simulink model "controller"  (R2019b)
settings: Solver=FixedStepDiscrete  StartTime=0.0  StopTime=10.0  FixedStep=0.01  RelTol=1e-3
settings Model: Creator=dommaschkj  LastModifiedBy=ReinfeldR
settings DataIOCC: ReturnWorkspaceOutputs=off
settings OptimizationCC: DefaultParameterBehavior=Inlined  UseDivisionForNetSlopeComputation=on  PassReuseOutputArgsAs=Individual arguments  MaxStackSize=64  EfficientTunableParamExpr=on
settings DebuggingCC: SignalInfNanChecking=warning  IntegerOverflowMsg=error  ParameterTunabilityLossMsg=error  AssertControl=DisableAll  SFUndirectedBroadcastEventsDiag=error  ArithmeticOperatorsInVariantConditions=warning
settings HardwareCC: ProdBitPerPointer=32  ProdBitPerSizeT=32  ProdBitPerPtrDiffT=32  ProdLargestAtomicInteger=LongLong  ProdLargestAtomicFloat=Double  ProdWordSize=32  ProdLongLongMode=on  ProdHWDeviceType=Custom Processor->Custom Processor
settings SFSimCC: SimUseLocalCustomCode=off  CompileTimeRecursionLimit=0  EnableRuntimeRecursion=off  MATLABDynamicMemAlloc=off  CustomCodeUndefinedFunction=UseInterfaceOnly
settings RTWCC: SystemTargetFile=ert.tlc  GenCodeOnly=on  PackageGeneratedCodeAndArtifacts=on  PackageName=controller  TemplateMakefile=ert_default_tmf  GenerateReport=on  RTWUseLocalCustomCode=off  Toolchain=GNU Tools for ARM Embedded Processors  IncludeHyperlinkInReport=on  LaunchReport=on  TargetLang=C++  GenerateTraceInfo=on  GenerateTraceReport=on  GenerateTraceReportSl=on  GenerateTraceReportSf=on  GenerateTraceReportEml=on
settings CodeAppCC: ForceParamTrailComments=on  IgnoreCustomStorageClasses=off  OperatorAnnotations=on  SimulinkDataObjDesc=on  SFDataObjDesc=on  MATLABFcnDesc=on  InsertBlockDesc=on
settings ERTTargetCC: TargetLangStandard=C99 (ISO)  UtilityFuncGeneration=Shared location  MultiwordLength=64  MultiInstanceERTCode=on  CodeInterfacePackaging=C++ class  SupportNonFinite=off  SupportComplex=off  ParenthesesLevel=Maximum  CastingMode=Standards  GenerateSharedConstants=off  InlinedParameterPlacement=NonHierarchical  RootIOFormat=Structure reference  ERTCustomFileTemplate=example_file_process.tlc  ERTFilePackagingFormat=Compact  EnableSignedLeftShifts=off  EnableSignedRightShifts=off

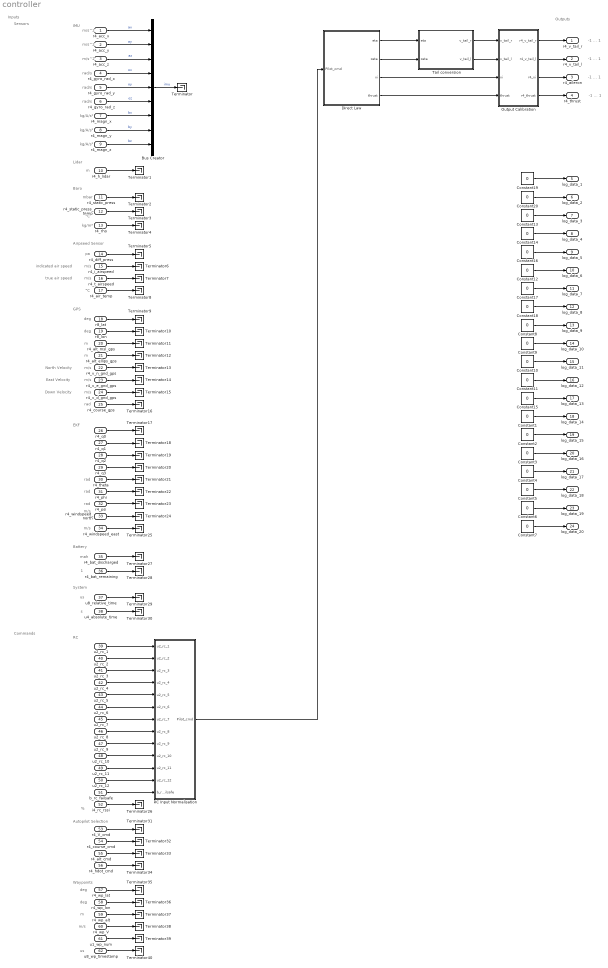
== system controller ==
  note: Sensors
  note: °C
  note: rad
  note: GPS
  note: IMU
  note: °C
  note: deg
  note: -1 ... 1
  note: Lidar
  note: -1 ... 1
  note: pa
  note: m
  note: m/s
  note: Down Velocity
  note: m
  note: North Velocity
  note: East Velocity
  note: m
  note: m/s^2
  note: Inputs
  note: -1 ... 1
  note: m/s
  note: -1 ... 1
  note: m/s
  note: m/s^2
  note: Outputs
  note: Airpseed Sensor
  note: mbar
  note: deg
  note: EKF
  note: rad
  note: Baro
  note: rad
  note: true air speed
  note: m/s^2
  note: rad
  note: m/s
  note: Battery
  note: kg/m³
  note: rad/s
  note: rad/s
  note: rad/s
  note: kg/A/s²
  note: kg/A/s²
  note: kg/A/s²
  note: m/s
  note: indicated air speed
  note: m/s
  note: m/s
  note: mah
  note: 1
  note: %
  note: us
  note: s
  note: System
  note: RC
  note: Commands
  note: Autopilot Selection
  note: Waypoints
  note: deg
  note: m
  note: m/s
  note: deg
  note: us
  r4_acc_x : Inport  OutDataTypeStr=single  Unit=m/s^2  PortDimensions=1  SampleTime=1/100  Interpolate=off
  r4_acc_y : Inport  Port=2  OutDataTypeStr=single  Unit=m/s^2  PortDimensions=1  SampleTime=1/100  Interpolate=off
  r4_acc_z : Inport  Port=3  OutDataTypeStr=single  Unit=m/s^2  PortDimensions=1  SampleTime=1/100  Interpolate=off
  r4_gyro_rad_x : Inport  Port=4  OutDataTypeStr=single  Unit=rad/s  PortDimensions=1  SampleTime=1/100  Interpolate=off
  r4_gyro_rad_y : Inport  Port=5  OutDataTypeStr=single  Unit=rad/s  PortDimensions=1  SampleTime=1/100  Interpolate=off
  r4_gyro_rad_z : Inport  Port=6  OutDataTypeStr=single  Unit=rad/s  PortDimensions=1  SampleTime=1/100  Interpolate=off  LockScale=on
  r4_magn_x : Inport  Port=7  OutDataTypeStr=single  Unit=kg/A/s^2  PortDimensions=1  SampleTime=1/100  Interpolate=off
  r4_magn_y : Inport  Port=8  OutDataTypeStr=single  Unit=kg/A/s^2  PortDimensions=1  SampleTime=1/100  Interpolate=off
  r4_magn_z : Inport  Port=9  OutDataTypeStr=single  Unit=kg/A/s^2  PortDimensions=1  SampleTime=1/100  Interpolate=off
  r4_h_lidar : Inport  Port=10  OutDataTypeStr=single  Unit=m  PortDimensions=1  SampleTime=1/100  Interpolate=off
  r4_static_press : Inport  Port=11  OutDataTypeStr=single  Unit=mbar  PortDimensions=1  SampleTime=1/100  Interpolate=off
  r4_static_press_temp : Inport  Port=12  OutDataTypeStr=single  Unit=°C  PortDimensions=1  SampleTime=1/100  Interpolate=off
  r4_rho : Inport  Port=13  OutDataTypeStr=single  Unit=kg/m^3  PortDimensions=1  SampleTime=1/100  Interpolate=off
  r4_diff_press : Inport  Port=14  OutDataTypeStr=single  Unit=Pa  PortDimensions=1  SampleTime=1/100  Interpolate=off
  r4_i_airspeed : Inport  Port=15  OutDataTypeStr=single  Unit=m/s  PortDimensions=1  SampleTime=1/100  Interpolate=off
  r4_t_airspeed : Inport  Port=16  OutDataTypeStr=single  Unit=m/s  PortDimensions=1  SampleTime=1/100  Interpolate=off
  r4_air_temp : Inport  Port=17  OutDataTypeStr=single  Unit=°C  PortDimensions=1  SampleTime=1/100  Interpolate=off
  r8_lat : Inport  Port=18  OutDataTypeStr=double  Unit=deg  PortDimensions=1  SampleTime=1/2  Interpolate=off
  r8_lon : Inport  Port=19  OutDataTypeStr=double  Unit=deg  PortDimensions=1  SampleTime=1/2  Interpolate=off
  r4_alt_msl_gps : Inport  Port=20  OutDataTypeStr=single  Unit=m  PortDimensions=1  SampleTime=1/2  Interpolate=off
  r4_alt_ellips_gps : Inport  Port=21  OutDataTypeStr=single  Unit=m  PortDimensions=1  SampleTime=1/2  Interpolate=off
  r4_v_n_gnd_gps : Inport  Port=22  OutDataTypeStr=single  Unit=m/s  PortDimensions=1  SampleTime=1/2  Interpolate=off
  r4_v_e_gnd_gps : Inport  Port=23  OutDataTypeStr=single  Unit=m/s  PortDimensions=1  SampleTime=1/2  Interpolate=off
  r4_v_d_gnd_gps : Inport  Port=24  OutDataTypeStr=single  Unit=m/s  PortDimensions=1  SampleTime=1/2  Interpolate=off
  r4_course_gps : Inport  Port=25  OutDataTypeStr=single  Unit=rad  PortDimensions=1  SampleTime=1/2  Interpolate=off
  r4_q0 : Inport  Port=26  OutMin=[-1]  OutMax=[1]  OutDataTypeStr=single  Unit=1  PortDimensions=1  SampleTime=1/100  Interpolate=off
  r4_q1 : Inport  Port=27  OutMin=[-1]  OutMax=[1]  OutDataTypeStr=single  Unit=1  PortDimensions=1  SampleTime=1/100  Interpolate=off
  r4_q2 : Inport  Port=28  OutMin=[-1]  OutMax=[1]  OutDataTypeStr=single  Unit=1  PortDimensions=1  SampleTime=1/100  Interpolate=off
  r4_q3 : Inport  Port=29  OutMin=[-1]  OutMax=[1]  OutDataTypeStr=single  Unit=one  PortDimensions=1  SampleTime=1/100  Interpolate=off
  r4_theta : Inport  Port=30  OutDataTypeStr=single  Unit=rad  PortDimensions=1  SampleTime=1/100  Interpolate=off
  r4_phi : Inport  Port=31  OutDataTypeStr=single  Unit=rad  PortDimensions=1  SampleTime=1/100  Interpolate=off
  r4_psi : Inport  Port=32  OutDataTypeStr=single  Unit=rad  PortDimensions=1  SampleTime=1/100  Interpolate=off
  r4_windspeed_north : Inport  Port=33  OutDataTypeStr=single  Unit=m/s  PortDimensions=1  SampleTime=1/100  Interpolate=off
  r4_windspeed_east : Inport  Port=34  OutDataTypeStr=single  Unit=m/s  PortDimensions=1  SampleTime=1/100  Interpolate=off
  r4_bat_discharged : Inport  Port=35  OutDataTypeStr=single  Unit=mA*hr  PortDimensions=1  SampleTime=1/100  Interpolate=off
  r4_bat_remaining : Inport  Port=36  OutDataTypeStr=single  PortDimensions=1  SampleTime=1/100  Interpolate=off
  u8_relative_time : Inport  Port=37  OutDataTypeStr=uint64  Unit=µs  PortDimensions=1  SampleTime=1/100  Interpolate=off
  u4_absolute_time : Inport  Port=38  OutDataTypeStr=uint32  Unit=s  PortDimensions=1  SampleTime=1/100  Interpolate=off
  u2_rc_1 : Inport  Port=39  OutDataTypeStr=uint16  PortDimensions=1  SampleTime=1/100  Interpolate=off
  u2_rc_2 : Inport  Port=40  OutDataTypeStr=uint16  PortDimensions=1  SampleTime=1/100  Interpolate=off
  u2_rc_3 : Inport  Port=41  OutDataTypeStr=uint16  PortDimensions=1  SampleTime=1/100  Interpolate=off
  u2_rc_4 : Inport  Port=42  OutDataTypeStr=uint16  PortDimensions=1  SampleTime=1/100  Interpolate=off
  u2_rc_5 : Inport  Port=43  OutDataTypeStr=uint16  PortDimensions=1  SampleTime=1/100  Interpolate=off
  u2_rc_6 : Inport  Port=44  OutDataTypeStr=uint16  PortDimensions=1  SampleTime=1/100  Interpolate=off
  u2_rc_7 : Inport  Port=45  OutDataTypeStr=uint16  PortDimensions=1  SampleTime=1/100  Interpolate=off
  u2_rc_8 : Inport  Port=46  OutDataTypeStr=uint16  PortDimensions=1  SampleTime=1/100  Interpolate=off
  u2_rc_9 : Inport  Port=47  OutDataTypeStr=uint16  PortDimensions=1  SampleTime=1/100  Interpolate=off
  u2_rc_10 : Inport  Port=48  OutDataTypeStr=uint16  PortDimensions=1  SampleTime=1/100  Interpolate=off
  u2_rc_11 : Inport  Port=49  OutDataTypeStr=uint16  PortDimensions=1  SampleTime=1/100  Interpolate=off
  u2_rc_12 : Inport  Port=50  OutDataTypeStr=uint16  PortDimensions=1  SampleTime=1/100  Interpolate=off
  b_rc_failsafe : Inport  Port=51  OutDataTypeStr=boolean  PortDimensions=1  SampleTime=1/100  Interpolate=off
  i4_rc_rssi : Inport  Port=52  OutDataTypeStr=int32  PortDimensions=1  SampleTime=1/100  Interpolate=off
  r4_V_cmd : Inport  Port=53  OutDataTypeStr=single  PortDimensions=1  SampleTime=1/100  Interpolate=off
  r4_course_cmd : Inport  Port=54  OutDataTypeStr=single  PortDimensions=1  SampleTime=1/100  Interpolate=off
  r4_alt_cmd : Inport  Port=55  OutDataTypeStr=single  PortDimensions=1  SampleTime=1/100  Interpolate=off
  r4_hdot_cmd : Inport  Port=56  OutDataTypeStr=single  PortDimensions=1  SampleTime=1/100  Interpolate=off
  r4_wp_lat : Inport  Port=57  OutDataTypeStr=single  Unit=deg  PortDimensions=15  SampleTime=1/100  Interpolate=off
  r4_wp_lon : Inport  Port=58  OutDataTypeStr=single  Unit=deg  PortDimensions=15  SampleTime=1/100  Interpolate=off
  r4_wp_alt : Inport  Port=59  OutDataTypeStr=single  Unit=m  PortDimensions=15  SampleTime=1/100  Interpolate=off
  r4_wp_V : Inport  Port=60  OutDataTypeStr=single  Unit=m/s  PortDimensions=15  SampleTime=1/100  Interpolate=off
  u1_wp_num : Inport  Port=61  OutDataTypeStr=uint8  PortDimensions=1  SampleTime=1/100  Interpolate=off
  u8_wp_timestamp : Inport  Port=62  OutMin=0  OutMax=18446744073709551615  OutDataTypeStr=uint64  Unit=µs  PortDimensions=1  SampleTime=1/100  Interpolate=off
  Bus Creator : BusCreator  Inputs=9
  Constant{1..20} (20 alike) : Constant  Value=0  OutDataTypeStr=single
  Direct Law : Subsystem
  Output Calibration : Subsystem
  RC Input Normalisation : Subsystem
  Tail conversion : Subsystem
  Terminator{,1..40} (41 alike) : Terminator
  r4_v_tail_r : Outport  OutDataTypeStr=single  VectorParamsAs1DForOutWhenUnconnected=off
  r4_v_tail_l : Outport  Port=2  OutDataTypeStr=single  VectorParamsAs1DForOutWhenUnconnected=off
  r4_aileron : Outport  Port=3  OutDataTypeStr=single  VectorParamsAs1DForOutWhenUnconnected=off
  r4_thrust : Outport  Port=4  OutDataTypeStr=single  VectorParamsAs1DForOutWhenUnconnected=off
  log_data_1 : Outport  Port=5  OutDataTypeStr=single  VectorParamsAs1DForOutWhenUnconnected=off
  log_data_2 : Outport  Port=6  OutDataTypeStr=single  VectorParamsAs1DForOutWhenUnconnected=off
  log_data_3 : Outport  Port=7  OutDataTypeStr=single  VectorParamsAs1DForOutWhenUnconnected=off
  log_data_4 : Outport  Port=8  OutDataTypeStr=single  VectorParamsAs1DForOutWhenUnconnected=off
  log_data_5 : Outport  Port=9  OutDataTypeStr=single  VectorParamsAs1DForOutWhenUnconnected=off
  log_data_6 : Outport  Port=10  OutDataTypeStr=single  VectorParamsAs1DForOutWhenUnconnected=off
  log_data_7 : Outport  Port=11  OutDataTypeStr=single  VectorParamsAs1DForOutWhenUnconnected=off
  log_data_8 : Outport  Port=12  OutDataTypeStr=single  VectorParamsAs1DForOutWhenUnconnected=off
  log_data_9 : Outport  Port=13  OutDataTypeStr=single  VectorParamsAs1DForOutWhenUnconnected=off
  log_data_10 : Outport  Port=14  OutDataTypeStr=single  VectorParamsAs1DForOutWhenUnconnected=off
  log_data_11 : Outport  Port=15  OutDataTypeStr=single  VectorParamsAs1DForOutWhenUnconnected=off
  log_data_12 : Outport  Port=16  OutDataTypeStr=single  VectorParamsAs1DForOutWhenUnconnected=off
  log_data_13 : Outport  Port=17  OutDataTypeStr=single  VectorParamsAs1DForOutWhenUnconnected=off
  log_data_14 : Outport  Port=18  OutDataTypeStr=single  VectorParamsAs1DForOutWhenUnconnected=off
  log_data_15 : Outport  Port=19  OutDataTypeStr=single  VectorParamsAs1DForOutWhenUnconnected=off
  log_data_16 : Outport  Port=20  OutDataTypeStr=single  VectorParamsAs1DForOutWhenUnconnected=off
  log_data_17 : Outport  Port=21  OutDataTypeStr=single  VectorParamsAs1DForOutWhenUnconnected=off
  log_data_18 : Outport  Port=22  OutDataTypeStr=single  VectorParamsAs1DForOutWhenUnconnected=off
  log_data_19 : Outport  Port=23  OutDataTypeStr=single  VectorParamsAs1DForOutWhenUnconnected=off
  log_data_20 : Outport  Port=24  OutDataTypeStr=single  VectorParamsAs1DForOutWhenUnconnected=off
  wires:
  Output Calibration/4(r4_thrust) -> r4_thrust/1
  Output Calibration/1(r4_v_tail_r) -> r4_v_tail_r/1
  Output Calibration/3(r4_xi) -> r4_aileron/1
  Output Calibration/2(r4_v_tail_l) -> r4_v_tail_l/1
  Tail conversion/1(v_tail_r) -> Output Calibration/1(v_tail_r)
  Tail conversion/2(v_tail_l) -> Output Calibration/2(v_tail_l)
  Direct Law/4(thrust) -> Output Calibration/4(thrust)
  u2_rc_1/1 -> RC Input Normalisation/1(u2_rc_1)
  u2_rc_2/1 -> RC Input Normalisation/2(u2_rc_2)
  u2_rc_3/1 -> RC Input Normalisation/3(u2_rc_3)
  u2_rc_4/1 -> RC Input Normalisation/4(u2_rc_4)
  u2_rc_5/1 -> RC Input Normalisation/5(u2_rc_5)
  u2_rc_7/1 -> RC Input Normalisation/7(u2_rc_7)
  u2_rc_8/1 -> RC Input Normalisation/8(u2_rc_8)
  u2_rc_6/1 -> RC Input Normalisation/6(u2_rc_6)
  b_rc_failsafe/1 -> RC Input Normalisation/13(b_rc_failsafe)
  Direct Law/3(xi) -> Output Calibration/3(xi)
  Direct Law/2(zeta) -> Tail conversion/2(zeta)
  Direct Law/1(eta) -> Tail conversion/1(eta)
  Bus Creator/1 -> Terminator/1  "imu"
  r4_acc_x/1 -> Bus Creator/1  "ax"
  r4_acc_y/1 -> Bus Creator/2  "ay"
  r4_acc_z/1 -> Bus Creator/3  "az"
  r4_gyro_rad_x/1 -> Bus Creator/4  "ox"
  r4_gyro_rad_y/1 -> Bus Creator/5  "oy"
  r4_gyro_rad_z/1 -> Bus Creator/6  "oz"
  r4_magn_x/1 -> Bus Creator/7  "bx"
  r4_magn_y/1 -> Bus Creator/8  "by"
  r4_magn_z/1 -> Bus Creator/9  "bz"
  r4_h_lidar/1 -> Terminator1/1
  r4_static_press/1 -> Terminator2/1
  r4_static_press_temp/1 -> Terminator3/1
  r4_rho/1 -> Terminator4/1
  r4_diff_press/1 -> Terminator5/1
  r4_i_airspeed/1 -> Terminator6/1
  r4_t_airspeed/1 -> Terminator7/1
  r4_air_temp/1 -> Terminator8/1
  r4_alt_msl_gps/1 -> Terminator11/1
  r4_alt_ellips_gps/1 -> Terminator12/1
  r4_v_n_gnd_gps/1 -> Terminator13/1
  r4_v_e_gnd_gps/1 -> Terminator14/1
  r4_v_d_gnd_gps/1 -> Terminator15/1
  r4_course_gps/1 -> Terminator16/1
  r4_q0/1 -> Terminator17/1
  r4_q1/1 -> Terminator18/1
  r4_q2/1 -> Terminator19/1
  r4_q3/1 -> Terminator20/1
  r4_theta/1 -> Terminator21/1
  r4_phi/1 -> Terminator22/1
  r4_psi/1 -> Terminator23/1
  r4_windspeed_north/1 -> Terminator24/1
  r4_windspeed_east/1 -> Terminator25/1
  i4_rc_rssi/1 -> Terminator26/1
  r4_bat_discharged/1 -> Terminator27/1
  r4_bat_remaining/1 -> Terminator28/1
  u8_relative_time/1 -> Terminator29/1
  u4_absolute_time/1 -> Terminator30/1
  u2_rc_9/1 -> RC Input Normalisation/9(u2_rc_9)
  u2_rc_10/1 -> RC Input Normalisation/10(u2_rc_10)
  u2_rc_11/1 -> RC Input Normalisation/11(u2_rc_11)
  u2_rc_12/1 -> RC Input Normalisation/12(u2_rc_12)
  RC Input Normalisation/1(Pilot_cmd) -> Direct Law/1(Pilot_cmd)
  Constant10/1 -> log_data_11/1
  Constant11/1 -> log_data_12/1
  Constant8/1 -> log_data_9/1
  Constant9/1 -> log_data_10/1
  r4_alt_cmd/1 -> Terminator33/1
  r4_course_cmd/1 -> Terminator32/1
  r4_hdot_cmd/1 -> Terminator34/1
  r4_V_cmd/1 -> Terminator31/1
  Constant15/1 -> log_data_13/1
  Constant2/1 -> log_data_15/1
  Constant4/1 -> log_data_17/1
  Constant1/1 -> log_data_14/1
  Constant5/1 -> log_data_18/1
  Constant7/1 -> log_data_20/1
  Constant3/1 -> log_data_16/1
  Constant6/1 -> log_data_19/1
  Constant20/1 -> log_data_2/1
  Constant14/1 -> log_data_4/1
  Constant18/1 -> log_data_8/1
  Constant19/1 -> log_data_1/1
  Constant17/1 -> log_data_7/1
  Constant13/1 -> log_data_3/1
  Constant12/1 -> log_data_6/1
  Constant16/1 -> log_data_5/1
  r8_lat/1 -> Terminator9/1
  r8_lon/1 -> Terminator10/1
  r4_wp_alt/1 -> Terminator37/1
  r4_wp_V/1 -> Terminator38/1
  r4_wp_lat/1 -> Terminator35/1
  r4_wp_lon/1 -> Terminator36/1
  u8_wp_timestamp/1 -> Terminator40/1
  u1_wp_num/1 -> Terminator39/1

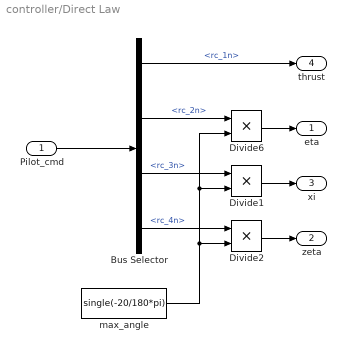
== system controller/Direct Law ==
  Pilot_cmd : Inport
  Bus Selector : BusSelector  OutputSignals=rc_1n,rc_2n,rc_3n,rc_4n
  Divide1 : Product  Inputs=**
  Divide2 : Product  Inputs=**
  Divide6 : Product  Inputs=**
  max_angle : Constant  Value=single(-20/180*pi)
  eta : Outport
  zeta : Outport  Port=2
  xi : Outport  Port=3
  thrust : Outport  Port=4
  wires:
  Pilot_cmd/1 -> Bus Selector/1
  Bus Selector/1 -> thrust/1  "<rc_1n>"
  Bus Selector/2 -> Divide6/1  "<rc_2n>"
  Bus Selector/4 -> Divide2/1  "<rc_4n>"
  Bus Selector/3 -> Divide1/1  "<rc_3n>"
  Divide6/1 -> eta/1
  Divide1/1 -> xi/1
  Divide2/1 -> zeta/1
  max_angle/1 -> Divide2/2, Divide1/2, Divide6/2

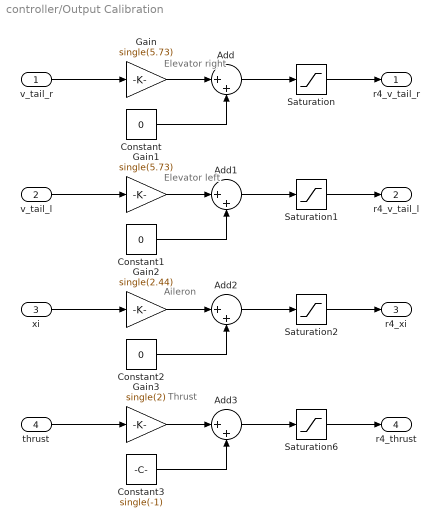
== system controller/Output Calibration ==
  note: Elevator right
  note: Elevator left
  note: Aileron
  note: Thrust
  v_tail_r : Inport  OutDataTypeStr=single  Unit=rad
  v_tail_l : Inport  Port=2  Unit=rad
  xi : Inport  Port=3  Unit=rad
  thrust : Inport  Port=4  Unit=1
  Add{,1..3} (4 alike) : Sum  Inputs=|++  InputSameDT=on  OutDataTypeStr=Inherit: Same as first input
  Constant : Constant  Value=0  OutDataTypeStr=single
  Constant1 : Constant  Value=0  OutDataTypeStr=single
  Constant2 : Constant  Value=0  OutDataTypeStr=single
  Constant3 : Constant  Value=single(-1)  OutDataTypeStr=single
  Gain : Gain  Gain=single(5.73)  OutDataTypeStr=single
  Gain1 : Gain  Gain=single(5.73)  OutDataTypeStr=single
  Gain2 : Gain  Gain=single(2.44)  OutDataTypeStr=single
  Gain3 : Gain  Gain=single(2)  OutDataTypeStr=single
  Saturation{,1..2,6} (4 alike) : Saturate  UpperLimit=1  LowerLimit=-1  OutDataTypeStr=single
  r4_v_tail_r : Outport  OutDataTypeStr=single  VectorParamsAs1DForOutWhenUnconnected=off
  r4_v_tail_l : Outport  Port=2  VectorParamsAs1DForOutWhenUnconnected=off
  r4_xi : Outport  Port=3  VectorParamsAs1DForOutWhenUnconnected=off
  r4_thrust : Outport  Port=4  VectorParamsAs1DForOutWhenUnconnected=off
  wires:
  v_tail_r/1 -> Gain/1
  Add/1 -> Saturation/1
  Saturation/1 -> r4_v_tail_r/1
  Gain/1 -> Add/1
  Constant/1 -> Add/2
  Gain1/1 -> Add1/1
  Saturation1/1 -> r4_v_tail_l/1
  v_tail_l/1 -> Gain1/1
  Add1/1 -> Saturation1/1
  Constant1/1 -> Add1/2
  Gain2/1 -> Add2/1
  Saturation2/1 -> r4_xi/1
  xi/1 -> Gain2/1
  Add2/1 -> Saturation2/1
  Constant2/1 -> Add2/2
  Saturation6/1 -> r4_thrust/1
  Gain3/1 -> Add3/1
  Constant3/1 -> Add3/2
  thrust/1 -> Gain3/1
  Add3/1 -> Saturation6/1

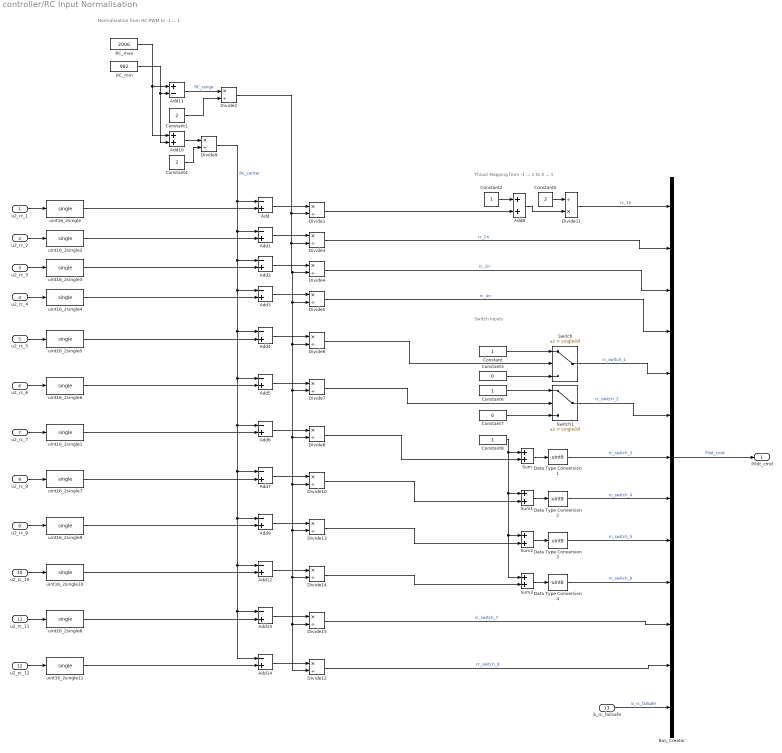
== system controller/RC Input Normalisation ==
  note: Thrust Mapping from -1 ... 1 to 0 ... 1
  note: Normalisation from RC PWM to -1 ... 1
  note: Switch Inputs
  u2_rc_1 : Inport  OutMin=0  OutMax=65535  OutDataTypeStr=uint16  Unit=1  PortDimensions=1  SampleTime=1/100
  u2_rc_2 : Inport  Port=2  OutMin=0  OutMax=65535  OutDataTypeStr=uint16  Unit=1  PortDimensions=1  SampleTime=1/100
  u2_rc_3 : Inport  Port=3  OutMin=0  OutMax=65535  OutDataTypeStr=uint16  Unit=1  PortDimensions=1  SampleTime=1/100
  u2_rc_4 : Inport  Port=4  OutMin=0  OutMax=65535  OutDataTypeStr=uint16  Unit=1  PortDimensions=1  SampleTime=1/100
  u2_rc_5 : Inport  Port=5  OutMin=0  OutMax=65535  OutDataTypeStr=uint16  Unit=1  PortDimensions=1  SampleTime=1/100
  u2_rc_6 : Inport  Port=6  OutMin=0  OutMax=65535  OutDataTypeStr=uint16  Unit=1  PortDimensions=1  SampleTime=1/100
  u2_rc_7 : Inport  Port=7  OutMin=0  OutMax=65535  OutDataTypeStr=uint16  Unit=1  PortDimensions=1  SampleTime=1/100
  u2_rc_8 : Inport  Port=8  OutMin=0  OutMax=65535  OutDataTypeStr=uint16  Unit=1  PortDimensions=1  SampleTime=1/100
  u2_rc_9 : Inport  Port=9  OutMin=0  OutMax=65535  OutDataTypeStr=uint16  Unit=1  PortDimensions=1  SampleTime=1/100
  u2_rc_10 : Inport  Port=10  OutMin=0  OutMax=65535  OutDataTypeStr=uint16  Unit=1  PortDimensions=1  SampleTime=1/100
  u2_rc_11 : Inport  Port=11  OutMin=0  OutMax=65535  OutDataTypeStr=uint16  Unit=1  PortDimensions=1  SampleTime=1/100
  u2_rc_12 : Inport  Port=12  OutMin=0  OutMax=65535  OutDataTypeStr=uint16  Unit=1  PortDimensions=1  SampleTime=1/100
  b_rc_failsafe : Inport  Port=13  OutMin=0  OutMax=1  OutDataTypeStr=boolean  Unit=1  PortDimensions=1  SampleTime=1/100
  Add{,1..7,9,12..14} (12 alike) : Sum  Inputs=-+  OutDataTypeStr=single
  Add10 : Sum
  Add11 : Sum  Inputs=+-
  Add8 : Sum  OutDataTypeStr=single
  Bus_Creator : BusCreator  Inputs=13
  Constant : Constant  OutDataTypeStr=uint8
  Constant1 : Constant  Value=2  OutDataTypeStr=single
  Constant2 : Constant  OutDataTypeStr=single
  Constant3 : Constant  Value=0  OutDataTypeStr=uint8
  Constant4 : Constant  Value=2  OutDataTypeStr=single
  Constant5 : Constant  Value=2  OutDataTypeStr=single
  Constant6 : Constant  OutDataTypeStr=uint8
  Constant7 : Constant  Value=0  OutDataTypeStr=uint8
  Constant8 : Constant  OutDataTypeStr=single
  Data Type Conversion{1..4} (4 alike) : DataTypeConversion  OutDataTypeStr=uint8  RndMeth=Nearest
  Divide{1..10,12..15} (14 alike) : Product  Inputs=*/
  Divide11 : Product  Inputs=/*
  RC_max : Constant  Value=2006  OutDataTypeStr=int16
  RC_min : Constant  Value=982  OutDataTypeStr=int16
  Sum{,1..3} (4 alike) : Sum
  Switch : Switch  Criteria=u2 > Threshold  Threshold=single(0)
  Switch1 : Switch  Criteria=u2 > Threshold  Threshold=single(0)
  uint16_2single{,1..11} (12 alike) : DataTypeConversion  OutDataTypeStr=single
  Pilot_cmd : Outport  VectorParamsAs1DForOutWhenUnconnected=off
  wires:
  uint16_2single5/1 -> Add4/2
  u2_rc_4/1 -> uint16_2single4/1
  u2_rc_2/1 -> uint16_2single2/1
  u2_rc_3/1 -> uint16_2single3/1
  u2_rc_1/1 -> uint16_2single/1
  Bus_Creator/1 -> Pilot_cmd/1  "Pilot_cmd"
  u2_rc_6/1 -> uint16_2single6/1
  Divide4/1 -> Bus_Creator/3  "rc_3n"
  RC_max/1 -> Add10/1, Add11/1
  Divide5/1 -> Bus_Creator/4  "rc_4n"
  u2_rc_5/1 -> uint16_2single5/1
  RC_min/1 -> Add10/2, Add11/2
  uint16_2single3/1 -> Add2/2
  uint16_2single/1 -> Add/2
  Divide3/1 -> Bus_Creator/2  "rc_2n"
  uint16_2single4/1 -> Add3/2
  uint16_2single2/1 -> Add1/2
  Add10/1 -> Divide9/1
  Constant4/1 -> Divide9/2
  Add11/1 -> Divide2/1  "RC_range"
  u2_rc_7/1 -> uint16_2single1/1
  u2_rc_8/1 -> uint16_2single7/1
  uint16_2single1/1 -> Add6/2
  uint16_2single7/1 -> Add7/2
  uint16_2single6/1 -> Add5/2
  Constant1/1 -> Divide2/2
  Add/1 -> Divide1/1
  Add1/1 -> Divide3/1
  Add2/1 -> Divide4/1
  Add3/1 -> Divide5/1
  Add4/1 -> Divide6/1
  Add5/1 -> Divide7/1
  Add6/1 -> Divide8/1
  Add7/1 -> Divide10/1
  Divide1/1 -> Add8/2
  Constant2/1 -> Add8/1
  Constant5/1 -> Divide11/1
  Add8/1 -> Divide11/2
  Constant/1 -> Switch/1
  Constant3/1 -> Switch/3
  Constant6/1 -> Switch1/1
  Constant7/1 -> Switch1/3
  Divide6/1 -> Switch/2
  Divide7/1 -> Switch1/2
  Divide11/1 -> Bus_Creator/1  "rc_1n"
  Switch/1 -> Bus_Creator/5  "rc_switch_1"
  Switch1/1 -> Bus_Creator/6  "rc_switch_2"
  b_rc_failsafe/1 -> Bus_Creator/13  "b_rc_failsafe"
  Divide8/1 -> Sum/2
  Sum/1 -> Data Type Conversion1/1
  Constant8/1 -> Sum3/1, Sum2/1, Sum1/1, Sum/1
  uint16_2single11/1 -> Add14/2
  Add14/1 -> Divide12/1
  u2_rc_10/1 -> uint16_2single10/1
  u2_rc_11/1 -> uint16_2single8/1
  u2_rc_12/1 -> uint16_2single11/1
  Add12/1 -> Divide14/1
  uint16_2single10/1 -> Add12/2
  Add13/1 -> Divide15/1
  u2_rc_9/1 -> uint16_2single9/1
  Divide9/1 -> Add14/1, Add13/1, Add12/1, Add9/1, Add7/1, Add6/1, Add5/1, Add4/1, Add3/1, Add2/1, Add1/1, Add/1  "RC_center"
  uint16_2single8/1 -> Add13/2
  Add9/1 -> Divide13/1
  uint16_2single9/1 -> Add9/2
  Divide2/1 -> Divide12/2, Divide15/2, Divide14/2, Divide13/2, Divide10/2, Divide8/2, Divide7/2, Divide6/2, Divide5/2, Divide4/2, Divide3/2, Divide1/2
  Divide10/1 -> Sum1/2
  Divide13/1 -> Sum2/2
  Divide14/1 -> Sum3/2
  Divide15/1 -> Bus_Creator/11  "rc_switch_7"
  Divide12/1 -> Bus_Creator/12  "rc_switch_8"
  Sum3/1 -> Data Type Conversion4/1
  Sum2/1 -> Data Type Conversion3/1
  Sum1/1 -> Data Type Conversion2/1
  Data Type Conversion1/1 -> Bus_Creator/7  "rc_switch_3"
  Data Type Conversion2/1 -> Bus_Creator/8  "rc_switch_4"
  Data Type Conversion3/1 -> Bus_Creator/9  "rc_switch_5"
  Data Type Conversion4/1 -> Bus_Creator/10  "rc_switch_6"

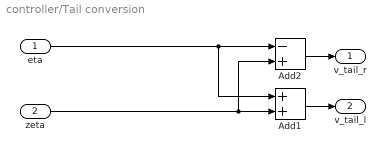
== system controller/Tail conversion ==
  eta : Inport  Unit=rad
  zeta : Inport  Port=2  Unit=rad
  Add1 : Sum
  Add2 : Sum  Inputs=-+
  v_tail_r : Outport  Unit=rad
  v_tail_l : Outport  Port=2  Unit=rad
  wires:
  zeta/1 -> Add2/2, Add1/2
  eta/1 -> Add2/1, Add1/1
  Add1/1 -> v_tail_l/1
  Add2/1 -> v_tail_r/1
